simulink model "A16_PD_Lageregelung_Regelstrecke"  (R2017b)
settings: Solver=ode45  StartTime=0.0  StopTime=4  MaxStep=1E-1  RelTol=1e-3  EnableMultiTasking=on
values from neighbouring files (symbols this model uses):
  CM = 7.1e-7    (= 7.1e-07)    [A10_Konstanten.m]    (also in A13_Konstanten.m; A14_Konstanten.m; A16_Konstanten.m)
  JL = 2e-4    (= 0.0002)    [A10_Konstanten.m]    (also in A16_Konstanten.m)
  JR = 1.32e-6    (= 1.32e-06)    [A10_Konstanten.m]    (also in A13_Konstanten.m; A14_Konstanten.m; A16_Konstanten.m; A9_Konstanten.m = 0.004)
  KM = 38.4e-3    (= 0.0384)    [A10_Konstanten.m]    (also in A13_Konstanten.m; A14_Konstanten.m; A16_Konstanten.m)
  KN = 1/(2*pi*KM)    (= 4.14465997635)    [A10_Konstanten.m]    (also in A13_Konstanten.m; A14_Konstanten.m; A16_Konstanten.m)
  LA = 4.64e-4    (= 0.000464)    [A10_Konstanten.m]    (also in A13_Konstanten.m; A14_Konstanten.m; A16_Konstanten.m)
  MW = 0    [A10_Konstanten.m]    (also in A16_Konstanten.m = 0.001)
  n0 = 10    [A16_Konstanten.m]
  R = 0.02    [A10_Konstanten.m]    (also in A13_Konstanten.m = 0.04; A14_Konstanten.m = 0.04; A16_Konstanten.m)
  RA = 4.99    [A10_Konstanten.m]    (also in A13_Konstanten.m; A14_Konstanten.m; A16_Konstanten.m)
settings Model: Creator=jbaur  LastModifiedBy=jbaur
settings DataIOCC: ExternalInput=X1  SaveFormat=StructureWithTime  SignalLoggingName=sigsOut
settings OptimizationCC: ExpressionDepthLimit=2147483647  InitFltsAndDblsToZero=on  LifeSpan=inf
settings DebuggingCC: SaveWithParameterizedLinksMsg=none  SignalResolutionControl=TryResolveAllWithWarning  MultiTaskDSMMsg=warning  MultiTaskCondExecSysMsg=none  StateNameClashWarn=warning  SFUnexpectedBacktrackingDiag=warning  SFNoUnconditionalDefaultTransitionDiag=warning  SFExecutionAtInitializationDiag=none
settings HardwareCC: ProdBitPerPointer=32  ProdBitPerSizeT=32  ProdBitPerPtrDiffT=32  ProdLargestAtomicFloat=None  ProdIntDivRoundTo=Undefined  ProdEndianess=Unspecified  ProdWordSize=32  ProdHWDeviceType=32-bit Generic  TargetUnknown=on
settings ModelReferenceCC: PropagateSignalLabelsOutOfModel=off
settings CodeAppCC: StateflowObjectComments=on
settings GRTTargetCC: TargetFcnLib=ansi_tfl_tmw.mat  TargetLangStandard=C89/C90 (ANSI)  ModelReferenceCompliant=off  GeneratePreprocessorConditionals=Disable all  CombineOutputUpdateFcns=off  MatFileLogging=off  GRTInterface=on
settings ConfigComp: CovMetricSettings=dw  CovHtmlReporting=on  CovSaveCumulativeToWorkspaceVar=on  CovSaveSingleToWorkspaceVar=on  CovExternalEMLEnable=off  CovSFcnEnable=off

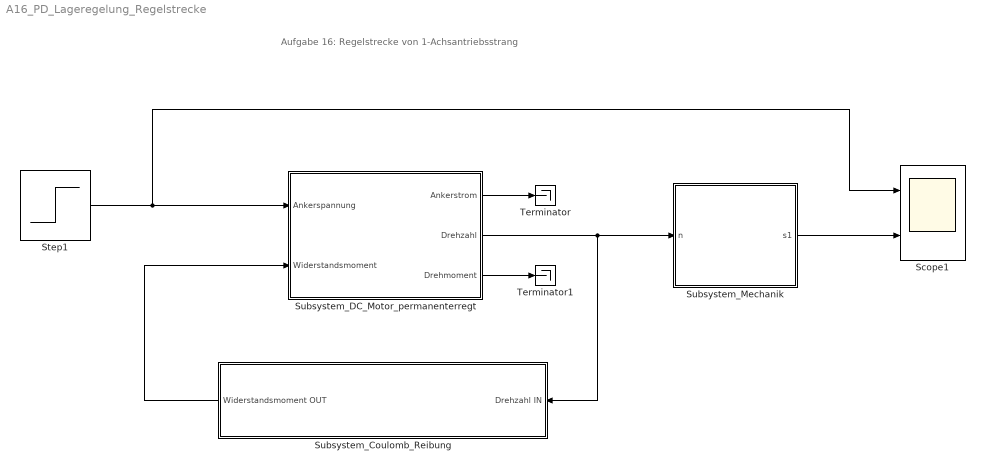
== system A16_PD_Lageregelung_Regelstrecke ==
  note: Aufgabe 16: Regelstrecke von 1-Achsantriebsstrang
  Scope1 : Scope  NumInputPorts=2
  Step1 : Step  Time=0  SampleTime=0
  Subsystem_Coulomb_Reibung : Subsystem
  Subsystem_DC_Motor_permanenterregt : Subsystem
  Subsystem_Mechanik : Subsystem
  Terminator : Terminator
  Terminator1 : Terminator
  wires:
  Step1/1 -> Scope1/1, Subsystem_DC_Motor_permanenterregt/1(Ankerspannung)
  Subsystem_Mechanik/1(s1) -> Scope1/2
  Subsystem_DC_Motor_permanenterregt/2(Drehzahl) -> Subsystem_Coulomb_Reibung/1(Drehzahl IN), Subsystem_Mechanik/1(n)
  Subsystem_Coulomb_Reibung/1(Widerstandsmoment OUT) -> Subsystem_DC_Motor_permanenterregt/2(Widerstandsmoment)
  Subsystem_DC_Motor_permanenterregt/3(Drehmoment) -> Terminator1/1
  Subsystem_DC_Motor_permanenterregt/1(Ankerstrom) -> Terminator/1

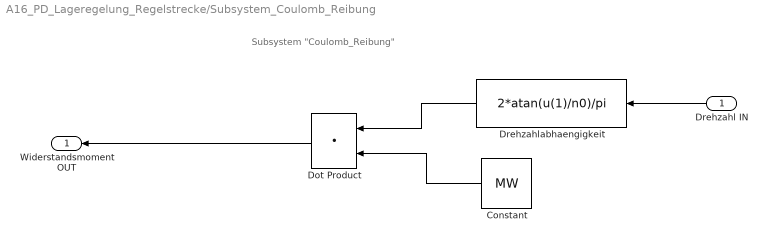
== system A16_PD_Lageregelung_Regelstrecke/Subsystem_Coulomb_Reibung ==
  note: Subsystem "Coulomb_Reibung"
  Drehzahl IN : Inport
  Constant : Constant  Value=MW
  Dot Product : DotProduct  InputSameDT=on  OutDataTypeStr=Inherit: Inherit via internal rule
  Drehzahlabhaengigkeit : Fcn  Expr=2*atan(u(1)/n0)/pi
  Widerstandsmoment OUT : Outport
  wires:
  Drehzahl IN/1 -> Drehzahlabhaengigkeit/1
  Drehzahlabhaengigkeit/1 -> Dot Product/1
  Constant/1 -> Dot Product/2
  Dot Product/1 -> Widerstandsmoment OUT/1

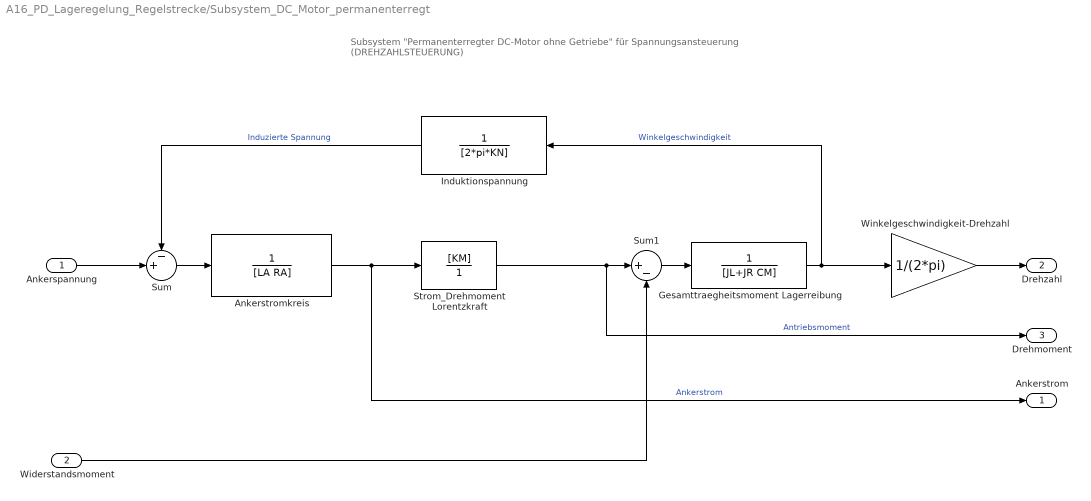
== system A16_PD_Lageregelung_Regelstrecke/Subsystem_DC_Motor_permanenterregt ==
  note: Subsystem "Permanenterregter DC-Motor ohne Getriebe"
      | für Spannungsansteuerung (DREHZAHLSTEUERUNG)
  Ankerspannung : Inport
  Widerstandsmoment : Inport  Port=2
  Ankerstromkreis : TransferFcn  Denominator=[LA RA]
  Gesamttraegheitsmoment Lagerreibung : TransferFcn  Denominator=[JL+JR CM]
  Induktionspannung : TransferFcn  Denominator=[2*pi*KN]
  Strom_Drehmoment Lorentzkraft : TransferFcn  Numerator=[KM]  Denominator=[1]
  Sum : Sum  Inputs=-+|
  Sum1 : Sum  Inputs=|+-
  Winkelgeschwindigkeit-Drehzahl : Gain  Gain=1/(2*pi)
  Ankerstrom : Outport
  Drehzahl : Outport  Port=2
  Drehmoment : Outport  Port=3
  wires:
  Ankerspannung/1 -> Sum/2
  Sum/1 -> Ankerstromkreis/1
  Induktionspannung/1 -> Sum/1  "Induzierte Spannung"
  Gesamttraegheitsmoment Lagerreibung/1 -> Induktionspannung/1, Winkelgeschwindigkeit-Drehzahl/1  "Winkelgeschwindigkeit"
  Strom_Drehmoment Lorentzkraft/1 -> Sum1/1, Drehmoment/1  "Antriebsmoment"
  Sum1/1 -> Gesamttraegheitsmoment Lagerreibung/1
  Ankerstromkreis/1 -> Ankerstrom/1, Strom_Drehmoment Lorentzkraft/1  "Ankerstrom"
  Winkelgeschwindigkeit-Drehzahl/1 -> Drehzahl/1
  Widerstandsmoment/1 -> Sum1/2

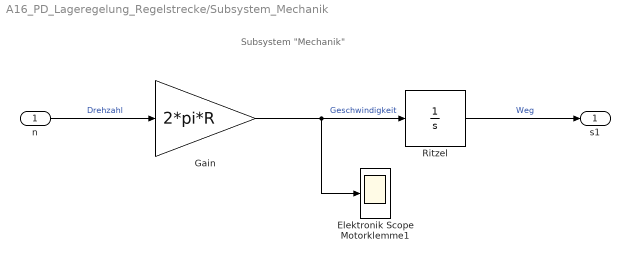
== system A16_PD_Lageregelung_Regelstrecke/Subsystem_Mechanik ==
  note: Subsystem "Mechanik"
  n : Inport
  Elektronik Scope Motorklemme1 : Scope
  Gain : Gain  Gain=2*pi*R
  Ritzel : TransferFcn  Denominator=[1 0]
  s1 : Outport
  wires:
  Ritzel/1 -> s1/1  "Weg"
  n/1 -> Gain/1  "Drehzahl"
  Gain/1 -> Elektronik Scope Motorklemme1/1, Ritzel/1  "Geschwindigkeit"
